simulink library "elementsLibrary"  (R2018a)
settings: Solver=VariableStepAuto  StartTime=0.0  StopTime=10.0  RelTol=1e-3
undefined symbols (not defined in the file): aerodynamics, ascent, avionics, environment, payload, propulsion, pvessel, recovery, rocket, sequencer
libraries: snippetLibrary x43, $bdroot x24, sharedutil x8, theirs_elementsLibrary x3, simulink_extras x1, aerolibutil x1
(part 1 of 4)
settings Model: Creator=Manit  LastModifiedBy=rohan

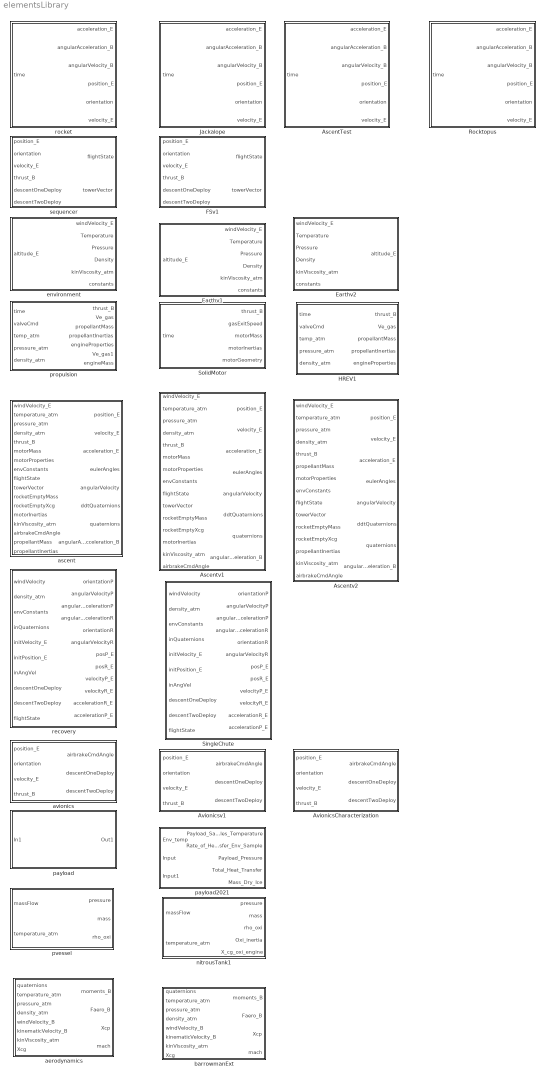
== system elementsLibrary ==
  AscentTest : Subsystem  mask{rocket=rocket}
      settings: MinAlgLoopOccurrences=on
  Ascentv1 : Subsystem  mask{ascent=ascent}
  Ascentv2 : Subsystem  mask{ascent=ascent}
  AvionicsCharacterization : Subsystem  mask{avionics=avionics}
  Avionicsv1 : Subsystem  mask{avionics=avionics}
  Earthv1 : Subsystem  mask{environment=environment}
  Earthv2 : Subsystem  mask{environment=environment}
  FSv1 : Subsystem  mask{sequencer=sequencer}
  HREV1 : Subsystem  mask{propulsion=propulsion}
  Jackalope : Subsystem  mask{rocket=rocket}
      settings: MinAlgLoopOccurrences=on
  Rocktopus : Subsystem  mask{rocket=rocket}
      settings: MinAlgLoopOccurrences=on
  SingleChute : Subsystem  mask{recovery=recovery}
  SolidMotor : Subsystem  mask{propulsion=propulsion}
  aerodynamics : Subsystem  BlockChoice=barrowmanExt
      settings: TemplateBlock=self  MemberBlocks=barrowmanExt
  ascent : Subsystem  BlockChoice=Ascentv1
      settings: TemplateBlock=self  MemberBlocks=Ascentv1,Ascentv2
  avionics : Subsystem  BlockChoice=Avionicsv1
      settings: TemplateBlock=self  MemberBlocks=AvionicsCharacterization,Avionicsv1
  barrowmanExt : Subsystem  mask{aerodynamics=aerodynamics}
  environment : Subsystem  BlockChoice=Earthv1
      settings: TemplateBlock=self  MemberBlocks=Earthv1,Earthv2
  nitrousTank1 : Subsystem  mask{pvessel=pvessel}
  payload : Subsystem  BlockChoice=payload2021
      settings: TemplateBlock=self  MemberBlocks=payload2021
  payload2021 : Subsystem  mask{payload=payload}
  propulsion : Subsystem  BlockChoice=HREV1
      settings: TemplateBlock=self  MemberBlocks=HREV1,SolidMotor
  pvessel : Subsystem  BlockChoice=nitrousTank1
      settings: TemplateBlock=self  MemberBlocks=nitrousTank1
  recovery : Subsystem  BlockChoice=SingleChute
      settings: TemplateBlock=self  MemberBlocks=SingleChute
  rocket : Subsystem  BlockChoice=Jackalope
      settings: TemplateBlock=self  MemberBlocks=Jackalope
  sequencer : Subsystem  BlockChoice=FSv1
      settings: TemplateBlock=self  MemberBlocks=FSv1

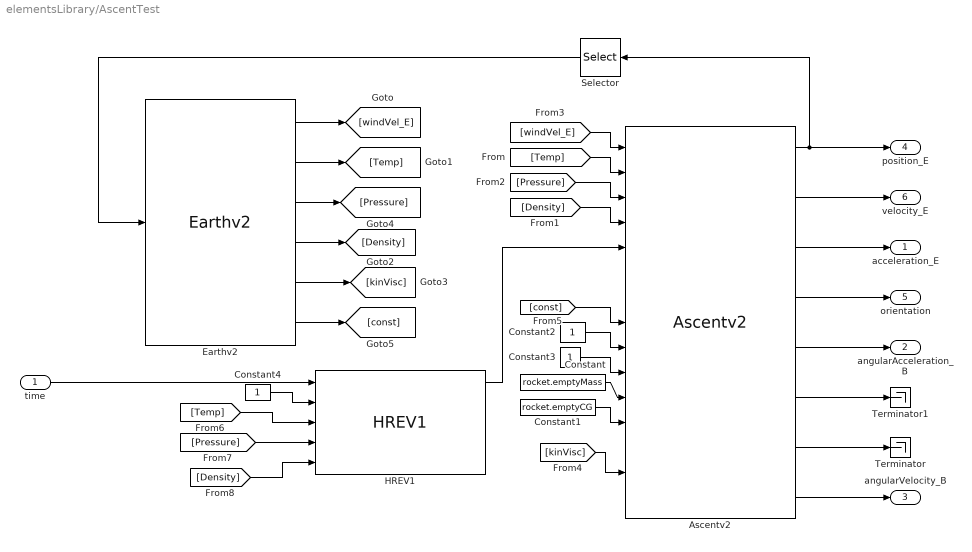
== system elementsLibrary/AscentTest ==
  time : Inport
  Ascentv2 : theirs_elementsLibrary/Ascentv2  ascent=ascent
  Constant : Constant  Value=rocket.emptyMass
  Constant1 : Constant  Value=rocket.emptyCG
  Constant2 : Constant
  Constant3 : Constant
  Constant4 : Constant
  Earthv2 : theirs_elementsLibrary/Earthv2  environment=environment
  HREV1 : theirs_elementsLibrary/HREV1  propulsion=propulsion
  Selector : Selector  InputPortWidth=3  IndexOptions=Index vector (dialog)  Indices=[3]  OutputSizes=1
  Terminator : Terminator
  Terminator1 : Terminator
  acceleration_E : Outport
  angularAcceleration_B : Outport  Port=2
  angularVelocity_B : Outport  Port=3
  position_E : Outport  Port=4
  orientation : Outport  Port=5
  velocity_E : Outport  Port=6
  wires:
  ? -> ?
  time/1 -> HREV1/1
  Ascentv2/1 -> position_E/1, Selector/1
  Selector/1 -> Earthv2/1
  Ascentv2/2 -> velocity_E/1
  Ascentv2/3 -> acceleration_E/1
  Ascentv2/5 -> angularAcceleration_B/1
  Ascentv2/8 -> angularVelocity_B/1
  Ascentv2/4 -> orientation/1
  Ascentv2/7 -> Terminator/1
  Ascentv2/6 -> Terminator1/1
  Earthv2/6 -> [const]
  Earthv2/5 -> [kinVisc]
  Earthv2/4 -> [Density]
  Earthv2/3 -> [Pressure]
  Earthv2/2 -> [Temp]
  Earthv2/1 -> [windVel_E]
  [windVel_E] -> Ascentv2/1
  [Temp] -> Ascentv2/2
  [Pressure] -> Ascentv2/3
  [Density] -> Ascentv2/4
  [const] -> Ascentv2/8
  [kinVisc] -> Ascentv2/14
  HREV1/1 -> Ascentv2/5
  [Temp] -> HREV1/3
  [Pressure] -> HREV1/4
  [Density] -> HREV1/5
  Constant/1 -> Ascentv2/11
  Constant1/1 -> Ascentv2/12
  Constant2/1 -> Ascentv2/9
  Constant3/1 -> Ascentv2/10
  Constant4/1 -> HREV1/2

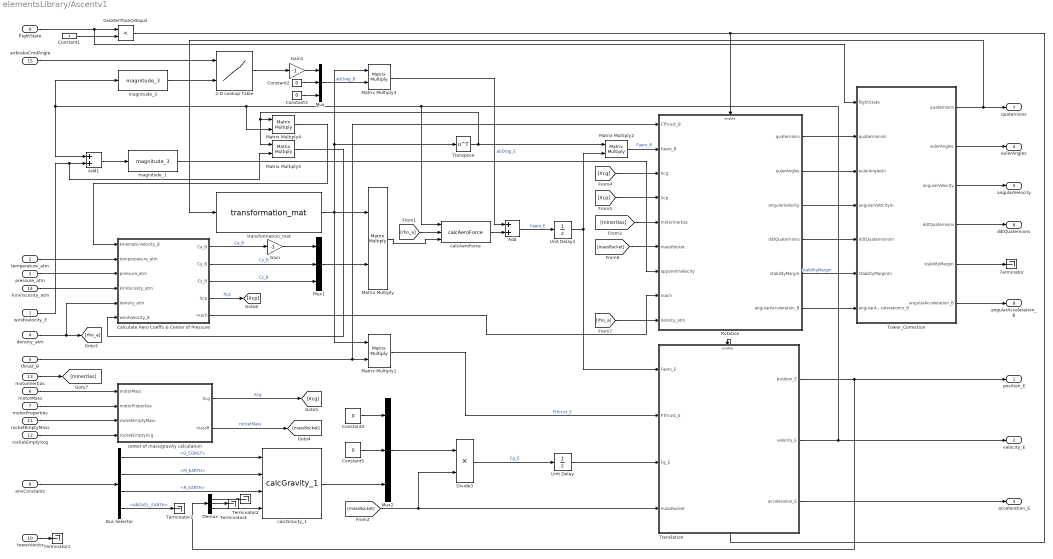
== system elementsLibrary/Ascentv1 ==
  windVelocity_E : Inport
  temperature_atm : Inport  Port=2
  pressure_atm : Inport  Port=3
  density_atm : Inport  Port=4
  thrust_B : Inport  Port=5
  motorMass : Inport  Port=6
  motorProperties : Inport  Port=7
  envConstants : Inport  Port=8
  flightState : Inport  Port=9
  towerVector : Inport  Port=10
  rocketEmptyMass : Inport  Port=11
  rocketEmptyXcg : Inport  Port=12
  motorInertias : Inport  Port=13
  kinViscosity_atm : Inport  Port=14
  airbrakeCmdAngle : Inport  Port=15
  2-D Lookup Table : Lookup_n-D  BreakpointsForDimension1=ascent.aerodynamics.cmdAngleBreakpoints  BreakpointsForDimension2=ascent.aerodynamics.speedBreakpoints  Table=ascent.aerodynamics.increaseInAxialDrag  ExtrapMethod=Clip  UseLastTableValue=on  InternalRulePriority=Speed  RndMeth=Simplest  InputSameDT=on
  Add : Sum
  Add1 : Sum
  Bus Selector : BusSelector  OutputSignals=G_CONST,M_EARTH,R_EARTH,ANGVEL_EARTH
  Calculate Aero Coeffs & Center of Pressure : Subsystem
  Constant1 : Constant  Value=4
  Constant{2..5} (4 alike) : Constant  Value=0
  Demux : Demux  Outputs=3
  Divide3 : Product  Inputs=**
  Gain : Gain  Gain=-1
  Gain1 : Gain  Gain=-1
  GreaterThanOrEqual : RelationalOperator  Operator=<  OutDataTypeStr=boolean  RndMeth=Simplest
  Matrix Multiply{,1..5} (6 alike) : Product  Multiplication=Matrix(*)
  Mux : Mux  Inputs=3
  Mux1 : Mux  Inputs=3
  Mux2 : Mux  Inputs=3
  Rotation : Subsystem
      settings: MinAlgLoopOccurrences=on
  Terminator{,1..4} (5 alike) : Terminator
  Tower_Correction : Subsystem
  Translation : Subsystem
  Transpose : Math  Operator=transpose  SaturateOnIntegerOverflow=on
  Unit Delay : UnitDelay  SampleTime=-1
  Unit Delay1 : UnitDelay  SampleTime=-1
  calcAeroForce : snippetLibrary/aeroSnippets/calcAeroForce  Aref=ascent.aerodynamics.Ar
  calcGravity_1 : snippetLibrary/dynamicsSnippets/calcGravity_1
  center of mass/gravity calculation : Subsystem
  magnitude_1 : snippetLibrary/mathSnippets/magnitude_3
  magnitude_3 : snippetLibrary/mathSnippets/magnitude_3
  transformation_mat : snippetLibrary/mathSnippets/transformation_mat
  position_E : Outport
  velocity_E : Outport  Port=2
  acceleration_E : Outport  Port=3
  eulerAngles : Outport  Port=4
  angularVelocity : Outport  Port=5
  ddtQuaternions : Outport  Port=6
  quaternions : Outport  Port=7
  angularAcceleration_B : Outport  Port=8
  wires:
  pressure_atm/1 -> Calculate Aero Coeffs & Center of Pressure/3(pressure_atm)
  temperature_atm/1 -> Calculate Aero Coeffs & Center of Pressure/2(temperpature_atm)
  density_atm/1 -> Calculate Aero Coeffs & Center of Pressure/5(density_atm), [rho_a]
  windVelocity_E/1 -> Matrix Multiply5/2, Add1/2
  Translation/2(velocity_E) -> velocity_E/1, Matrix Multiply4/2, magnitude_3/1, Add1/1, calcAeroForce/1
  envConstants/1 -> Bus Selector/1
  Bus Selector/4 -> Terminator3/1  "<ANGVEL_EARTH>"
  Bus Selector/1 -> calcGravity_1/1  "<G_CONST>"
  Bus Selector/2 -> calcGravity_1/2  "<M_EARTH>"
  Bus Selector/3 -> calcGravity_1/3  "<R_EARTH>"
  motorMass/1 -> center of mass/gravity calculation/1(motorMass)
  motorProperties/1 -> center of mass/gravity calculation/2(motorProperties)
  rocketEmptyMass/1 -> center of mass/gravity calculation/3(rocketEmptyMass)
  rocketEmptyXcg/1 -> center of mass/gravity calculation/4(rocketEmptyXcg)
  calcAeroForce/1 -> Add/2
  [rho_a] -> calcAeroForce/2
  transformation_mat/1 -> Matrix Multiply/1, Matrix Multiply1/1, Transpose/1, Matrix Multiply3/1
  Mux1/1 -> Matrix Multiply/2
  Matrix Multiply/1 -> calcAeroForce/3
  Calculate Aero Coeffs & Center of Pressure/1(Ca_B) -> Gain/1  "Ca_B"
  Gain/1 -> Mux1/1
  Calculate Aero Coeffs & Center of Pressure/2(Cy_B) -> Mux1/2  "Cy_B"
  Calculate Aero Coeffs & Center of Pressure/3(Cz_B) -> Mux1/3  "Cz_B"
  thrust_B/1 -> Rotation/1(FThrust_B), Matrix Multiply1/2
  Matrix Multiply1/1 -> Translation/2(FThrust_E)  "Fthrust_E"
  Divide3/1 -> Unit Delay/1  "Fg_E"
  Constant5/1 -> Mux2/2
  Mux2/1 -> Divide3/1
  calcGravity_1/1 -> Mux2/3
  Constant4/1 -> Mux2/1
  [massRocket] -> Divide3/2, Translation/4(massRocket)
  center of mass/gravity calculation/2(massR) -> [massRocket]  "rocketMass"
  center of mass/gravity calculation/1(Xcg) -> [Xcg]  "Xcg"
  Calculate Aero Coeffs & Center of Pressure/4(Xcp) -> [Xcp]  "Xcp"
  towerVector/1 -> Terminator1/1
  motorInertias/1 -> [mInertias]
  [mInertias] -> Rotation/5(motorInertias)
  [Xcg] -> Rotation/3(Xcg)
  [Xcp] -> Rotation/4(Xcp)
  Demux/3 -> calcGravity_1/4
  Demux/1 -> Terminator2/1
  Demux/2 -> Terminator4/1
  Matrix Multiply2/1 -> Rotation/2(Faero_B)  "Faero_B"
  Transpose/1 -> Matrix Multiply5/1, Matrix Multiply4/1, Matrix Multiply2/1
  [massRocket] -> Rotation/6(massRocket)
  Rotation/1(quaternions) -> Tower_Correction/2(quaternionsIn)
  airbrakeCmdAngle/1 -> 2-D Lookup Table/1
  flightState/1 -> Tower_Correction/1(flightState), GreaterThanOrEqual/1
  Constant1/1 -> GreaterThanOrEqual/2
  GreaterThanOrEqual/1 -> Rotation/Enable, Translation/Enable
  Mux/1 -> Matrix Multiply3/2  "abDrag_B"
  Constant2/1 -> Mux/2
  Constant3/1 -> Mux/3
  2-D Lookup Table/1 -> Gain1/1
  Gain1/1 -> Mux/1
  magnitude_3/1 -> 2-D Lookup Table/2
  Matrix Multiply3/1 -> Add/1  "abDrag_E"
  Add/1 -> Unit Delay1/1  "Faero_E"
  kinViscosity_atm/1 -> Calculate Aero Coeffs & Center of Pressure/4(kinViscosity_atm)
  Rotation/2(eulerAngles) -> Tower_Correction/3(eulerAnglesIn)
  Rotation/3(angularVelocity) -> Tower_Correction/4(angularVelocityIn)
  Rotation/4(ddtQuaternions) -> Tower_Correction/5(ddtQuaternionsIn)
  Rotation/5(stabilityMargin) -> Tower_Correction/6(stabilityMarginIn)  "stabilityMargin"
  Rotation/6(angularAcceleration_B) -> Tower_Correction/7(angularAccelerationIn_B)
  Translation/1(position_E) -> position_E/1, Demux/1
  Translation/3(acceleration_E) -> acceleration_E/1
  Tower_Correction/1(quaternions) -> quaternions/1, transformation_mat/1
  Tower_Correction/2(eulerAngles) -> eulerAngles/1
  Tower_Correction/3(angularVelocity) -> angularVelocity/1
  Tower_Correction/4(ddtQuaternions) -> ddtQuaternions/1
  Tower_Correction/5(stabilityMargin) -> Terminator/1
  Tower_Correction/6(angularAcceleration_B) -> angularAcceleration_B/1
  Unit Delay/1 -> Translation/3(Fg_E)
  Unit Delay1/1 -> Translation/1(Faero_E), Matrix Multiply2/2
  magnitude_1/1 -> Rotation/7(apparentVelocity)
  Calculate Aero Coeffs & Center of Pressure/5(mach) -> Rotation/8(mach)
  Add1/1 -> magnitude_1/1
  [rho_a] -> Rotation/9(density_atm)
  Matrix Multiply4/1 -> Calculate Aero Coeffs & Center of Pressure/1(kinematicVelocity_B)
  Matrix Multiply5/1 -> Calculate Aero Coeffs & Center of Pressure/6(windVelocity_B)

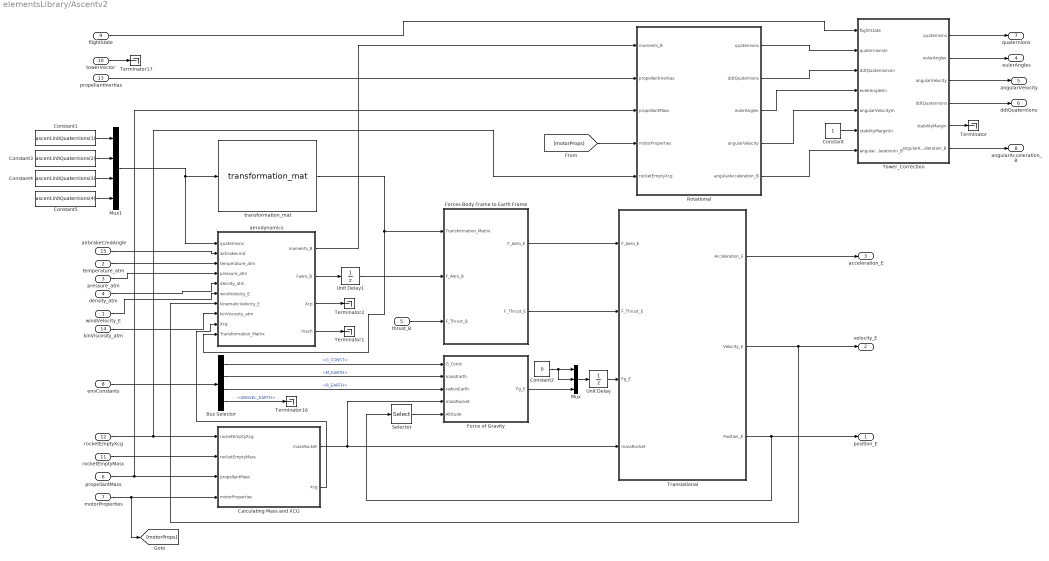
== system elementsLibrary/Ascentv2 ==
  windVelocity_E : Inport
  temperature_atm : Inport  Port=2
  pressure_atm : Inport  Port=3
  density_atm : Inport  Port=4
  thrust_B : Inport  Port=5
  propellantMass : Inport  Port=6
  motorProperties : Inport  Port=7
  envConstants : Inport  Port=8
  flightState : Inport  Port=9
  towerVector : Inport  Port=10
  rocketEmptyMass : Inport  Port=11
  rocketEmptyXcg : Inport  Port=12
  propellantInertias : Inport  Port=13
  kinViscosity_atm : Inport  Port=14
  airbrakeCmdAngle : Inport  Port=15
  Bus Selector : BusSelector  OutputSignals=G_CONST,M_EARTH,R_EARTH,ANGVEL_EARTH
  Calculating Mass and XCG : Subsystem
  Constant : Constant
  Constant1 : Constant  Value=ascent.initQuaternions(1)
  Constant2 : Constant  Value=0
  Constant3 : Constant  Value=ascent.initQuaternions(2)
  Constant4 : Constant  Value=ascent.initQuaternions(3)
  Constant5 : Constant  Value=ascent.initQuaternions(4)
  Force of Gravity : Subsystem
  Forces Body Frame to Earth Frame : Subsystem
  Mux : Mux  Inputs=3
  Mux1 : Mux
  Rotational : Subsystem
  Selector : Selector  InputPortWidth=3  IndexOptions=Index vector (dialog)  Indices=[3]  OutputSizes=1
  Terminator{,1..2,16..17} (5 alike) : Terminator
  Tower_Correction : Subsystem
  "Translational " : Subsystem
  Unit Delay : UnitDelay  SampleTime=-1
  Unit Delay1 : UnitDelay  SampleTime=-1
  aerodynamics : Subsystem
  transformation_mat : snippetLibrary/mathSnippets/transformation_mat
  position_E : Outport
  velocity_E : Outport  Port=2
  acceleration_E : Outport  Port=3
  eulerAngles : Outport  Port=4
  angularVelocity : Outport  Port=5
  ddtQuaternions : Outport  Port=6
  quaternions : Outport  Port=7
  angularAcceleration_B : Outport  Port=8
  wires:
  Force of Gravity/1(Fg_E) -> Mux/3
  thrust_B/1 -> Forces Body Frame to Earth Frame/3(F_Thrust_B)
  Bus Selector/3 -> Force of Gravity/3(radiusEarth)  "<R_EARTH>"
  propellantMass/1 -> Calculating Mass and XCG/3(propellantMass), Rotational/3(propellantMass)
  Constant2/1 -> Mux/1, Mux/2
  rocketEmptyXcg/1 -> Calculating Mass and XCG/1(rocketEmptyXcg), Rotational/5(rocketEmptyXcg)
  Calculating Mass and XCG/1(massRocket) -> Force of Gravity/4(massRocket), "Translational "/4(massRocket)
  Forces Body Frame to Earth Frame/2(F_Thrust_E) -> "Translational "/2(F_Thrust_E)
  towerVector/1 -> Terminator17/1
  Bus Selector/4 -> Terminator16/1  "<ANGVEL_EARTH>"
  flightState/1 -> Tower_Correction/1(flightState)
  Bus Selector/2 -> Force of Gravity/2(massEarth)  "<M_EARTH>"
  rocketEmptyMass/1 -> Calculating Mass and XCG/2(rocketEmptyMass)
  pressure_atm/1 -> aerodynamics/4(pressure_atm)
  Selector/1 -> Force of Gravity/5(Altitude)
  Forces Body Frame to Earth Frame/1(F_Aero_E) -> "Translational "/1(F_Aero_E)
  motorProperties/1 -> [motorProps], Calculating Mass and XCG/4(motorProperties)
  airbrakeCmdAngle/1 -> aerodynamics/2(airbrakecmd)
  Bus Selector/1 -> Force of Gravity/1(G_Const)  "<G_CONST>"
  "Translational "/1(Acceleration_E) -> acceleration_E/1
  envConstants/1 -> Bus Selector/1
  propellantInertias/1 -> Rotational/2(propellentInertias)
  "Translational "/3(Position_E) -> position_E/1, Selector/1
  Calculating Mass and XCG/2(Xcg) -> aerodynamics/9(Xcg)
  "Translational "/2(Velocity_E) -> velocity_E/1, aerodynamics/7(kinematicVelocity_E)
  transformation_mat/1 -> Forces Body Frame to Earth Frame/1(Transformation_Matrix), aerodynamics/10(Transformation_Matrix)
  kinViscosity_atm/1 -> aerodynamics/8(kinViscosity_atm)
  windVelocity_E/1 -> aerodynamics/6(windVelocity_E)
  density_atm/1 -> aerodynamics/5(density_atm)
  temperature_atm/1 -> aerodynamics/3(temperature_atm)
  aerodynamics/1(moments_B) -> Rotational/1(moments_B)
  aerodynamics/3(Xcp) -> Terminator2/1
  aerodynamics/4(mach) -> Terminator1/1
  [motorProps] -> Rotational/4(motorProperties)
  Mux/1 -> Unit Delay/1
  Unit Delay/1 -> "Translational "/3(Fg_E)
  aerodynamics/2(Faero_B) -> Unit Delay1/1
  Unit Delay1/1 -> Forces Body Frame to Earth Frame/2(F_Aero_B)
  Constant/1 -> Tower_Correction/6(stabilityMarginIn)
  Rotational/5(angularAcceleration_B) -> Tower_Correction/7(angularAccelerationIn_B)
  Rotational/4(angularVelocity) -> Tower_Correction/5(angularVelocityIn)
  Rotational/3(eulerAngles) -> Tower_Correction/4(eulerAnglesIn)
  Rotational/2(ddtQuaternions) -> Tower_Correction/3(ddtQuaternionsIn)
  Tower_Correction/6(angularAcceleration_B) -> angularAcceleration_B/1
  Tower_Correction/3(angularVelocity) -> angularVelocity/1
  Tower_Correction/4(ddtQuaternions) -> ddtQuaternions/1
  Tower_Correction/2(eulerAngles) -> eulerAngles/1
  Tower_Correction/1(quaternions) -> quaternions/1
  Tower_Correction/5(stabilityMargin) -> Terminator/1
  Rotational/1(quaternions) -> Tower_Correction/2(quaternionsIn)
  Constant5/1 -> Mux1/4
  Constant3/1 -> Mux1/2
  Constant1/1 -> Mux1/1
  Constant4/1 -> Mux1/3
  Mux1/1 -> transformation_mat/1, aerodynamics/1(quaternions)

== system elementsLibrary/AvionicsCharacterization ==
  position_E : Inport
  orientation : Inport  Port=2
  velocity_E : Inport  Port=3
  thrust_B : Inport  Port=4
  Constant : Constant  Value=avionics.airbrakeDeploySpeed
  Constant1 : Constant  Value=avionics.airbrakeDeployCmd
  Constant2 : Constant  Value=avionics.descentTwoDeployAltitude
  Demux1 : Demux  Outputs=3
  Demux2 : Demux  Outputs=3
  MATLAB Function : MATLAB Function  TreatAsAtomicUnit=on
  Terminator{1..5} (5 alike) : Terminator
  Unit Delay : UnitDelay  InitialCondition=false  SampleTime=-1
  Unit Delay1 : UnitDelay  InitialCondition=false  SampleTime=-1
  Unit Delay2 : UnitDelay  InitialCondition=false  SampleTime=-1
  magnitude_1 : snippetLibrary/mathSnippets/magnitude_3
  magnitude_3 : snippetLibrary/mathSnippets/magnitude_3
  airbrakeCmdAngle : Outport
  descentOneDeploy : Outport  Port=2
  descentTwoDeploy : Outport  Port=3
  wires:
  thrust_B/1 -> magnitude_3/1
  velocity_E/1 -> Demux2/1, magnitude_1/1
  orientation/1 -> Terminator1/1
  position_E/1 -> Demux1/1
  MATLAB Function/1(airbrakeCmdAngle) -> Unit Delay2/1  "airbrakeCmdAngle"
  MATLAB Function/2(deploy1) -> Unit Delay1/1  "descentOneDeploy"
  MATLAB Function/3(deploy2) -> Unit Delay/1  "descentTwoDeploy"
  magnitude_1/1 -> MATLAB Function/2(velMag)
  Demux1/3 -> MATLAB Function/1(posZ_E)
  Demux1/1 -> Terminator2/1
  Demux1/2 -> Terminator3/1
  Constant/1 -> MATLAB Function/5(airbrakeDeploySpeed)
  Constant1/1 -> MATLAB Function/6(airbrakeDeployCmd)
  Constant2/1 -> MATLAB Function/7(descentTwoDeployAltitude)
  Demux2/3 -> MATLAB Function/3(velZ_E)
  Demux2/1 -> Terminator4/1
  Demux2/2 -> Terminator5/1
  Unit Delay/1 -> MATLAB Function/9(prevDeploy2), descentTwoDeploy/1
  magnitude_3/1 -> MATLAB Function/4(thurstMag_B)
  Unit Delay1/1 -> MATLAB Function/8(prevDeploy1), descentOneDeploy/1
  Unit Delay2/1 -> airbrakeCmdAngle/1

== system elementsLibrary/Avionicsv1 ==
  position_E : Inport
  orientation : Inport  Port=2
  velocity_E : Inport  Port=3
  thrust_B : Inport  Port=4
  airbrakeCmdAngle : Outport
  descentOneDeploy : Outport  Port=2
  descentTwoDeploy : Outport  Port=3

== system elementsLibrary/Earthv1 ==
  altitude_E : Inport
  1-D Lookup Table : Lookup_n-D  NumberOfTableDimensions=1  BreakpointsForDimension1=environment.altiBreakpoints  Table=environment.dynamicViscosityAir  ExtrapMethod=Clip  UseLastTableValue=on  InternalRulePriority=Speed  RndMeth=Simplest  InputSameDT=on
  Abs : Abs
  Bus Creator : BusCreator  Inputs=4
  Constant : Constant  Value=environment.RADIUS_EARTH
  Constant1 : Constant  Value=environment.MASS_EARTH
  Constant2 : Constant  Value=environment.ANGULARVELOCITY_EARTH
  Constant3 : Constant  Value=environment.GRAVITATION_CONST
  Constant4 : Constant  Value=0
  Cos : Trigonometry  Operator=cos
  Divide : Product  Inputs=/*
  MATLAB Function : MATLAB Function  TreatAsAtomicUnit=on
  Multiply : Product
  Multiply1 : Product
  Mux : Mux  Inputs=3
  Sin : Trigonometry
  Terminator : Terminator
  Wind Velocity Calculation : Subsystem
  encoded wind direction : Constant  Value=environment.referenceWindAngle
  windVelocity_E : Outport
  Temperature : Outport  Port=2
  Pressure : Outport  Port=3
  Density : Outport  Port=4
  kinViscosity_atm : Outport  Port=5
  constants : Outport  Port=6
  wires:
  MATLAB Function/3(density) -> Divide/1, Density/1  "atmos_density"
  MATLAB Function/2(pressure) -> Pressure/1  "atmos_pressure"
  Wind Velocity Calculation/1(Out1) -> Multiply1/1, Multiply/1  "windspeed"
  altitude_E/1 -> Wind Velocity Calculation/1(In1), Wind Velocity Calculation/2(Altitude), 1-D Lookup Table/1, MATLAB Function/1(altitude)
  MATLAB Function/1(temperature) -> Temperature/1  "atmos_temperature"
  Constant/1 -> Bus Creator/1  "R_EARTH"
  Constant1/1 -> Bus Creator/2  "M_EARTH"
  Constant2/1 -> Bus Creator/3  "ANGVEL_EARTH"
  Constant3/1 -> Bus Creator/4  "G_CONST"
  encoded wind direction/1 -> [windAngle]
  Multiply1/1 -> Mux/2
  Multiply/1 -> Mux/1
  Constant4/1 -> Mux/3
  Mux/1 -> Abs/1  "windvelocity_E"
  [windAngle] -> Sin/1, Cos/1
  Cos/1 -> Multiply/2
  Sin/1 -> Multiply1/2
  Bus Creator/1 -> constants/1
  1-D Lookup Table/1 -> Terminator/1, Divide/2  "dynamicViscosity"
  Divide/1 -> kinViscosity_atm/1  "kinViscosity"
  Abs/1 -> windVelocity_E/1

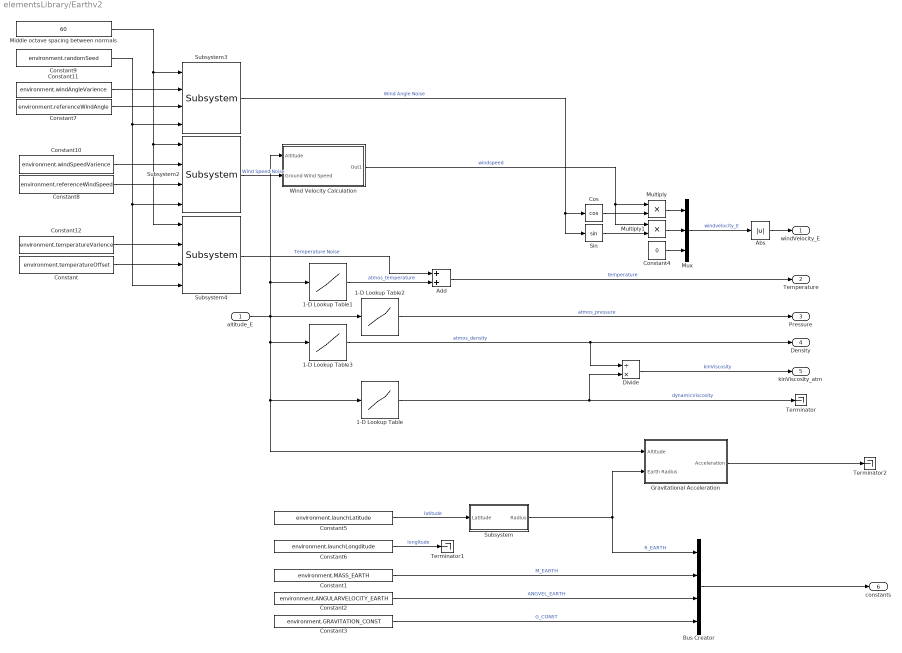
== system elementsLibrary/Earthv2 ==
  altitude_E : Inport
  1-D Lookup Table : Lookup_n-D  NumberOfTableDimensions=1  BreakpointsForDimension1=environment.altiBreakpoints  Table=environment.dynamicViscosityAir  ExtrapMethod=Clip  UseLastTableValue=on  InternalRulePriority=Speed  RndMeth=Simplest  InputSameDT=on
  1-D Lookup Table1 : Lookup_n-D  NumberOfTableDimensions=1  BreakpointsForDimension1=environment.altiBreakpoints  Table=environment.temperatureAir  ExtrapMethod=Clip  UseLastTableValue=on  InternalRulePriority=Speed  RndMeth=Simplest  InputSameDT=on
  1-D Lookup Table2 : Lookup_n-D  NumberOfTableDimensions=1  BreakpointsForDimension1=environment.altiBreakpoints  Table=environment.pressureAir  ExtrapMethod=Clip  UseLastTableValue=on  InternalRulePriority=Speed  RndMeth=Simplest  InputSameDT=on
  1-D Lookup Table3 : Lookup_n-D  NumberOfTableDimensions=1  BreakpointsForDimension1=environment.altiBreakpoints  Table=environment.densityAir  ExtrapMethod=Clip  UseLastTableValue=on  InternalRulePriority=Speed  RndMeth=Simplest  InputSameDT=on
  Abs : Abs
  Add : Sum
  Bus Creator : BusCreator  Inputs=4
  Constant : Constant  Value=environment.temperatureOffset
  Constant1 : Constant  Value=environment.MASS_EARTH
  Constant10 : Constant  Value=environment.windSpeedVarience
  Constant11 : Constant  Value=environment.windAngleVarience
  Constant12 : Constant  Value=environment.temperatureVarience
  Constant2 : Constant  Value=environment.ANGULARVELOCITY_EARTH
  Constant3 : Constant  Value=environment.GRAVITATION_CONST
  Constant4 : Constant  Value=0
  Constant5 : Constant  Value=environment.launchLatitude
  Constant6 : Constant  Value=environment.launchLongditude
  Constant7 : Constant  Value=environment.referenceWindAngle
  Constant8 : Constant  Value=environment.referenceWindSpeed
  Constant9 : Constant  Value=environment.randomSeed
  Cos : Trigonometry  Operator=cos
  Divide : Product  Inputs=/*
  Gravitational Acceleration : Subsystem
  Middle octave spacing between normals : Constant  Value=60
  Multiply : Product
  Multiply1 : Product
  Mux : Mux  Inputs=3
  Sin : Trigonometry
  Subsystem : Subsystem
  Subsystem2 : snippetLibrary/environmentSnippets/Subsystem
  Subsystem3 : snippetLibrary/environmentSnippets/Subsystem
  Subsystem4 : snippetLibrary/environmentSnippets/Subsystem
  Terminator : Terminator
  Terminator1 : Terminator
  Terminator2 : Terminator
  Wind Velocity Calculation : Subsystem
  windVelocity_E : Outport
  Temperature : Outport  Port=2
  Pressure : Outport  Port=3
  Density : Outport  Port=4
  kinViscosity_atm : Outport  Port=5
  constants : Outport  Port=6
  wires:
  Constant9/1 -> Subsystem4/4, Subsystem2/4, Subsystem3/4
  Constant12/1 -> Subsystem4/2
  Constant11/1 -> Subsystem3/2
  Constant10/1 -> Subsystem2/2
  Middle octave spacing between normals/1 -> Subsystem3/1, Subsystem2/1, Subsystem4/1
  Constant8/1 -> Subsystem2/3
  Constant7/1 -> Subsystem3/3
  Constant/1 -> Subsystem4/3
  Subsystem4/1 -> Add/1  "Temperature Noise"
  Subsystem3/1 -> Cos/1, Sin/1  "Wind Angle Noise"
  Subsystem2/1 -> Wind Velocity Calculation/2(Ground Wind Speed)  "Wind Speed Noise"
  Add/1 -> Temperature/1  "temperature"
  Subsystem/1(Radius) -> Gravitational Acceleration/2(Earth Radius), Bus Creator/1  "R_EARTH"
  Gravitational Acceleration/1(Acceleration) -> Terminator2/1
  Constant5/1 -> Subsystem/1(Latitude)  "latitude"
  Constant6/1 -> Terminator1/1  "longitude"
  altitude_E/1 -> 1-D Lookup Table3/1, 1-D Lookup Table/1, Gravitational Acceleration/1(Altitude), 1-D Lookup Table1/1, Wind Velocity Calculation/1(Altitude), 1-D Lookup Table2/1
  Abs/1 -> windVelocity_E/1
  Divide/1 -> kinViscosity_atm/1  "kinViscosity"
  1-D Lookup Table/1 -> Divide/2, Terminator/1  "dynamicViscosity"
  Bus Creator/1 -> constants/1
  Sin/1 -> Multiply1/2
  Cos/1 -> Multiply/2
  Mux/1 -> Abs/1  "windvelocity_E"
  Constant4/1 -> Mux/3
  Multiply/1 -> Mux/1
  Multiply1/1 -> Mux/2
  Constant3/1 -> Bus Creator/4  "G_CONST"
  Constant2/1 -> Bus Creator/3  "ANGVEL_EARTH"
  Constant1/1 -> Bus Creator/2  "M_EARTH"
  1-D Lookup Table1/1 -> Add/2  "atmos_temperature"
  Wind Velocity Calculation/1(Out1) -> Multiply/1, Multiply1/1  "windspeed"
  1-D Lookup Table2/1 -> Pressure/1  "atmos_pressure"
  1-D Lookup Table3/1 -> Density/1, Divide/1  "atmos_density"

== system elementsLibrary/FSv1 ==
  position_E : Inport
  orientation : Inport  Port=2
  velocity_E : Inport  Port=3
  thrust_B : Inport  Port=4
  descentOneDeploy : Inport  Port=5
  descentTwoDeploy : Inport  Port=6
  Demux1 : Demux  Outputs=3
  Demux2 : Demux  Outputs=3
  Demux4 : Demux  Outputs=3
  Length of Launch Tower1 : Constant  Value=sequencer.launchTower(1)
  Length of Launch Tower2 : Constant  Value=sequencer.launchTower(2)
  Length of Launch Tower3 : Constant  Value=sequencer.launchTower(3)
  MATLAB Function : MATLAB Function  TreatAsAtomicUnit=on
  Mux : Mux  Inputs=3
  Stop Simulation : Stop
  Unit Delay : UnitDelay  InitialCondition=sequencer.initialFlightState  SampleTime=-1
  magnitude3_1 : snippetLibrary/mathSnippets/magnitude_3
  magnitude3_3 : snippetLibrary/mathSnippets/magnitude_3
  magnitude_3 : snippetLibrary/mathSnippets/magnitude_3
  flightState : Outport
  towerVector : Outport  Port=2
  wires:
  position_E/1 -> magnitude3_1/1, Demux1/1
  MATLAB Function/1(flightState) -> Unit Delay/1  "flightState"
  thrust_B/1 -> magnitude_3/1
  Demux1/1 -> MATLAB Function/3(posX_E)
  Demux1/2 -> MATLAB Function/4(posY_E)
  Demux1/3 -> MATLAB Function/5(posZ_E)
  orientation/1 -> Demux2/1
  Length of Launch Tower1/1 -> Mux/1
  Length of Launch Tower2/1 -> Mux/2
  Length of Launch Tower3/1 -> Mux/3
  Mux/1 -> magnitude3_3/1, towerVector/1
  Demux2/2 -> MATLAB Function/7(pitch)
  Demux2/3 -> MATLAB Function/8(yaw)
  Demux2/1 -> MATLAB Function/6(roll)
  Unit Delay/1 -> MATLAB Function/15(prevFlightState), flightState/1
  magnitude3_1/1 -> MATLAB Function/2(posMag)
  Demux4/2 -> MATLAB Function/10(velY_E)
  Demux4/1 -> MATLAB Function/9(velX_E)
  Demux4/3 -> MATLAB Function/11(velZ_E)
  velocity_E/1 -> Demux4/1
  [towerLen] -> MATLAB Function/1(towerLen)
  magnitude_3/1 -> MATLAB Function/14(thurstMag_B)
  magnitude3_3/1 -> [towerLen]
  descentOneDeploy/1 -> MATLAB Function/12(descentOneDeploy)
  descentTwoDeploy/1 -> MATLAB Function/13(descentTwoDeploy)
  MATLAB Function/2(stop) -> Stop Simulation/1

== system elementsLibrary/HREV1 ==
  time : Inport
  valveCmd : Inport  Port=2
  temp_atm : Inport  Port=3
  pressure_atm : Inport  Port=4
  "density_atm " : Inport  Port=5
  Add1 : Sum
  Bus Creator : BusCreator  Inputs=2
  Chamber_Ballistics : Subsystem
  Injecter : Subsystem
  Nozzle : Subsystem
  Propellant_Mass : Subsystem
  Terminator{,1..8} (9 alike) : Terminator
  Unit Delay : UnitDelay  SampleTime=-1
  Unit Delay1 : UnitDelay  InitialCondition=101.325  SampleTime=-1
  X_grain_to_engine : Constant  Value=propulsion.X_TanktoGrain
  X_nose_to_engine : Constant  Value=propulsion.X_GM
  cg_propellent_engine : Subsystem
  nitrousTank1 : $bdroot/nitrousTank1  pvessel=propulsion.pvessel
  parallel_axis_propellent : Subsystem
  thrust_B : Outport
  Ve_gas : Outport  Port=2
  propellantMass : Outport  Port=3
  propellantInertias : Outport  Port=4
  engineProperties : Outport  Port=5
  wires:
  time/1 -> Terminator/1
  valveCmd/1 -> Terminator1/1
  pressure_atm/1 -> Nozzle/4(P_atm)
  Chamber_Ballistics/2(mdot_total) -> Nozzle/1(mdot)  "mdot_total"
  Chamber_Ballistics/3(Pc) -> Unit Delay1/1  "Pchamber"
  Chamber_Ballistics/4(Tc) -> Nozzle/3(Tc)  "Tchamber"
  Chamber_Ballistics/1(mdot_fuel) -> Terminator5/1  "mdot_fuel"
  Chamber_Ballistics/5(rdot_fuel) -> Terminator6/1  "rdot_fuel"
  nitrousTank1/2 -> Injecter/4(mass_oxi), cg_propellent_engine/4(mass_oxi), parallel_axis_propellent/1(mass_oxi), Propellant_Mass/1(mass_oxi)
  Chamber_Ballistics/6(massFlux_oxi) -> Terminator7/1  "Gox"
  Chamber_Ballistics/7(OF_ratio) -> Terminator8/1  "OF_ratio"
  Nozzle/4(charV) -> Unit Delay/1  "cStar"
  Unit Delay/1 -> Chamber_Ballistics/2(cStar)
  "density_atm "/1 -> Terminator3/1
  Nozzle/2(V_exit) -> Ve_gas/1  "Ve_gas"
  Nozzle/1(thrust_B) -> thrust_B/1  "thrust_B"
  Nozzle/3(mach_exit) -> Terminator4/1  "mach_exit"
  Propellant_Mass/1(massProp) -> propellantMass/1  "propellant_mass"
  Unit Delay1/1 -> Injecter/2(Chamber_pressure), Nozzle/2(Pc)
  Chamber_Ballistics/8(mass_fuel) -> cg_propellent_engine/2(mass_fuel), parallel_axis_propellent/6(mass_fuel), Propellant_Mass/2(mass_fuel)  "mass_fuel"
  X_grain_to_engine/1 -> Add1/2
  Chamber_Ballistics/10(X_cg_fuel) -> Add1/1
  Add1/1 -> cg_propellent_engine/1(X_cg_fuel_engine), parallel_axis_propellent/5(X_cg_fuel_engine)  "X_cg_fuel_engine"
  nitrousTank1/5 -> cg_propellent_engine/3(X_cg_oxi_engine), parallel_axis_propellent/3(X_cg_oxi_engine)
  cg_propellent_engine/1(cg_prop_engine) -> parallel_axis_propellent/8(X_cg_prop_engine), Bus Creator/2  "x_cg_B"
  parallel_axis_propellent/1(Propellent_inertia) -> propellantInertias/1
  nitrousTank1/4 -> parallel_axis_propellent/2(Oxi_inertia)
  Chamber_Ballistics/9(Fuel_inertia) -> parallel_axis_propellent/4(Fuel_inertia)
  X_nose_to_engine/1 -> Bus Creator/1, parallel_axis_propellent/7(X_nose_to_engine)  "x_gm_B"
  Bus Creator/1 -> engineProperties/1
  Injecter/1(mdot_oxi) -> nitrousTank1/1, Chamber_Ballistics/1(mdot_oxi)  "mdot_oxi"
  nitrousTank1/1 -> Injecter/1("Tank_pressure ")
  nitrousTank1/3 -> Injecter/3(density_oxi)
  temp_atm/1 -> nitrousTank1/2

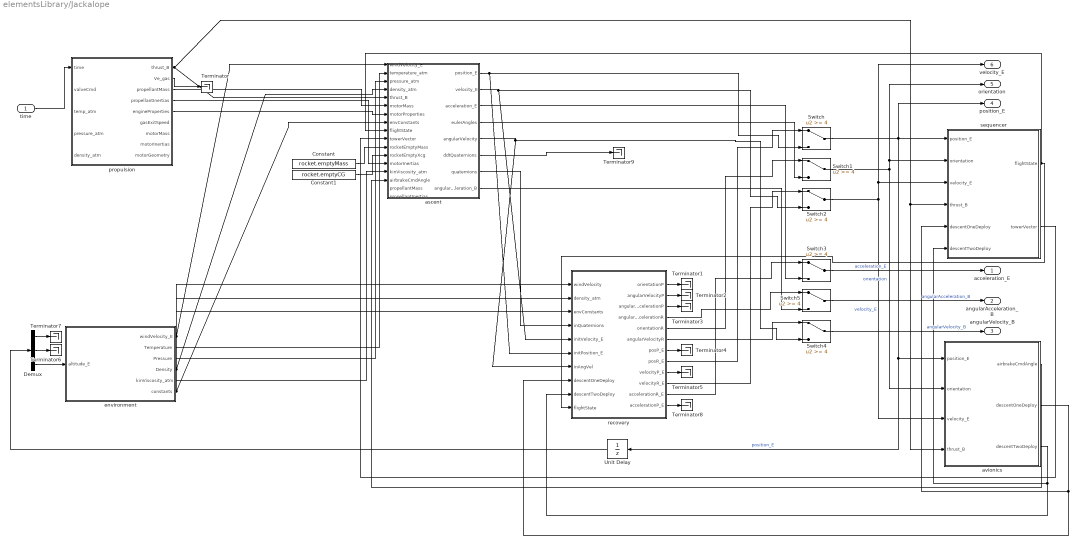
== system elementsLibrary/Jackalope ==
  time : Inport
  Constant : Constant  Value=rocket.emptyMass
  Constant1 : Constant  Value=rocket.emptyCG
  Demux : Demux  Outputs=3
  Switch{,1..5} (6 alike) : Switch  Threshold=4
  Terminator{,1..9} (10 alike) : Terminator
  Unit Delay : UnitDelay  SampleTime=-1
  ascent : Subsystem  BlockChoice=Ascentv1
      settings: AttributesFormatString=%<BlockChoice>  TemplateBlock=elementsLibrary/ascent  MemberBlocks=Ascentv1,Ascentv2
  avionics : Subsystem  BlockChoice=AvionicsCharacterization
      link override AvionicsCharacterization: avionics=rocket.avionics
      link override Avionicsv1: avionics=rocket.avionics
      settings: AttributesFormatString=%<BlockChoice>  TemplateBlock=elementsLibrary/avionics  MemberBlocks=AvionicsCharacterization,Avionicsv1
  environment : Subsystem  BlockChoice=Earthv1
      link override Earthv1: environment=rocket.environment
      settings: AttributesFormatString=%<BlockChoice>  TemplateBlock=elementsLibrary/environment  MemberBlocks=Earthv1,Earthv2
  propulsion : Subsystem  BlockChoice=SolidMotor
      link override SolidMotor: propulsion=rocket.propulsion
      settings: AttributesFormatString=%<BlockChoice>  TemplateBlock=elementsLibrary/propulsion  MemberBlocks=HREV1,SolidMotor
  recovery : Subsystem  BlockChoice=SingleChute
      link override SingleChute: recovery=rocket.recovery
      settings: AttributesFormatString=%<BlockChoice>  TemplateBlock=elementsLibrary/recovery  MemberBlocks=SingleChute
  sequencer : Subsystem  BlockChoice=FSv1
      link override FSv1: sequencer=rocket.sequencer
      settings: AttributesFormatString=%<BlockChoice>  TemplateBlock=elementsLibrary/sequencer  MemberBlocks=FSv1
  acceleration_E : Outport
  angularAcceleration_B : Outport  Port=2
  angularVelocity_B : Outport  Port=3
  position_E : Outport  Port=4
  orientation : Outport  Port=5
  velocity_E : Outport  Port=6
  wires:
  time/1 -> propulsion/1(time)
  Switch/1 -> sequencer/1(position_E), avionics/1(position_E), Unit Delay/1, position_E/1  "position_E"
  Switch1/1 -> avionics/2(orientation), sequencer/2(orientation), orientation/1  "orientation"
  Switch2/1 -> avionics/3(velocity_E), sequencer/3(velocity_E), velocity_E/1  "velocity_E"
  recovery/8(posR_E) -> Switch/1
  recovery/10(velocityR_E) -> Switch2/1
  ascent/4(eulerAngles) -> Switch1/3
  recovery/5(orientationR) -> Switch1/1
  environment/4(Density) -> ascent/4(density_atm), recovery/2(density_atm)
  environment/6(constants) -> ascent/8(envConstants), recovery/3(envConstants)
  environment/3(Pressure) -> ascent/3(pressure_atm)
  environment/2(Temperature) -> ascent/2(temperature_atm)
  environment/1(windVelocity_E) -> ascent/1(windVelocity_E), recovery/1(windVelocity)
  propulsion/3(propellantMass) -> ascent/6(motorMass)
  propulsion/4(propellantInertias) -> ascent/13(motorInertias)
  propulsion/1(thrust_B) -> ascent/5(thrust_B), sequencer/4(thrust_B), avionics/4(thrust_B)
  propulsion/5(engineProperties) -> ascent/7(motorProperties)
  propulsion/2(Ve_gas) -> Terminator/1
  sequencer/2(towerVector) -> ascent/10(towerVector)
  ascent/5(angularVelocity) -> recovery/7(inAngVel), Switch4/3
  ascent/1(position_E) -> Switch/3, recovery/6(initPosition_E)
  ascent/2(velocity_E) -> Switch2/3, recovery/5(initVelocity_E)
  recovery/2(angularVelocityP) -> Terminator2/1
  recovery/1(orientationP) -> Terminator1/1
  recovery/3(angularAccelerationP) -> Terminator3/1
  recovery/7(posP_E) -> Terminator4/1
  recovery/9(velocityP_E) -> Terminator5/1
  ascent/3(acceleration_E) -> Switch3/3
  ascent/7(quaternions) -> recovery/4(inQuaternions)
  Demux/3 -> environment/1(altitude_E)
  Demux/2 -> Terminator6/1
  Demux/1 -> Terminator7/1
  recovery/12(accelerationP_E) -> Terminator8/1
  recovery/11(accelerationR_E) -> Switch3/1
  Switch3/1 -> acceleration_E/1  "acceleration_E"
  recovery/4(angularAccelerationR) -> Switch5/1
  recovery/6(angularVelocityR) -> Switch4/1
  ascent/8(angularAcceleration_B) -> Switch5/3
  Switch5/1 -> angularAcceleration_B/1  "angularAcceleration_B"
  Switch4/1 -> angularVelocity_B/1  "angularVelocity_B"
  ascent/6(ddtQuaternions) -> Terminator9/1
  Constant/1 -> ascent/11(rocketEmptyMass)
  Constant1/1 -> ascent/12(rocketEmptyXcg)
  environment/5(kinViscosity_atm) -> ascent/14(kinViscosity_atm)
  avionics/3(descentTwoDeploy) -> recovery/9(descentTwoDeploy), sequencer/6(descentTwoDeploy)
  avionics/2(descentOneDeploy) -> sequencer/5(descentOneDeploy), recovery/8(descentOneDeploy)
  avionics/1(airbrakeCmdAngle) -> ascent/15(airbrakeCmdAngle)
  Unit Delay/1 -> Demux/1
  sequencer/1(flightState) -> ascent/9(flightState), recovery/10(flightState)

== system elementsLibrary/Rocktopus ==
  time : Inport
  Constant : Constant  Value=rocket.emptyMass
  Constant1 : Constant  Value=rocket.emptyCG
  Demux : Demux  Outputs=3
  Switch{,1..5} (6 alike) : Switch  Threshold=4
  Terminator{,1..9} (10 alike) : Terminator
  Unit Delay : UnitDelay  SampleTime=-1
  ascent : Subsystem  BlockChoice=Ascentv2
      link override Ascentv2: ascent=rocket.ascent
      settings: AttributesFormatString=%<BlockChoice>  TemplateBlock=elementsLibrary/ascent  MemberBlocks=Ascentv1,Ascentv2
  avionics : Subsystem  BlockChoice=AvionicsCharacterization
      link override AvionicsCharacterization: avionics=rocket.avionics
      link override Avionicsv1: avionics=rocket.avionics
      settings: AttributesFormatString=%<BlockChoice>  TemplateBlock=elementsLibrary/avionics  MemberBlocks=AvionicsCharacterization,Avionicsv1
  environment : Subsystem  BlockChoice=Earthv1
      link override Earthv1: environment=rocket.environment
      settings: AttributesFormatString=%<BlockChoice>  TemplateBlock=elementsLibrary/environment  MemberBlocks=Earthv1,Earthv2
  propulsion : Subsystem  BlockChoice=HREV1
      link override HREV1: propulsion=rocket.propulsion
      link override SolidMotor: propulsion=rocket.propulsion
      settings: AttributesFormatString=%<BlockChoice>  TemplateBlock=elementsLibrary/propulsion  MemberBlocks=HREV1,SolidMotor
  recovery : Subsystem  BlockChoice=SingleChute
      link override SingleChute: recovery=rocket.recovery
      settings: AttributesFormatString=%<BlockChoice>  TemplateBlock=elementsLibrary/recovery  MemberBlocks=SingleChute
  sequencer : Subsystem  BlockChoice=FSv1
      link override FSv1: sequencer=rocket.sequencer
      settings: AttributesFormatString=%<BlockChoice>  TemplateBlock=elementsLibrary/sequencer  MemberBlocks=FSv1
  acceleration_E : Outport
  angularAcceleration_B : Outport  Port=2
  angularVelocity_B : Outport  Port=3
  position_E : Outport  Port=4
  orientation : Outport  Port=5
  velocity_E : Outport  Port=6
  wires:
  time/1 -> propulsion/1(time)
  Switch/1 -> sequencer/1(position_E), avionics/1(position_E), Unit Delay/1, position_E/1  "position_E"
  Switch1/1 -> avionics/2(orientation), sequencer/2(orientation), orientation/1  "orientation"
  Switch2/1 -> avionics/3(velocity_E), sequencer/3(velocity_E), velocity_E/1  "velocity_E"
  recovery/8(posR_E) -> Switch/1
  recovery/10(velocityR_E) -> Switch2/1
  ascent/4(eulerAngles) -> Switch1/3
  recovery/5(orientationR) -> Switch1/1
  environment/4(Density) -> propulsion/5("density_atm "), ascent/4(density_atm), recovery/2(density_atm)
  environment/6(constants) -> ascent/8(envConstants), recovery/3(envConstants)
  environment/3(Pressure) -> propulsion/4(pressure_atm), ascent/3(pressure_atm)
  environment/2(Temperature) -> propulsion/3(temp_atm), ascent/2(temperature_atm)
  environment/1(windVelocity_E) -> ascent/1(windVelocity_E), recovery/1(windVelocity)
  propulsion/3(propellantMass) -> ascent/16(propellantMass)
  propulsion/1(thrust_B) -> ascent/5(thrust_B), sequencer/4(thrust_B), avionics/4(thrust_B)
  propulsion/5(engineProperties) -> ascent/7(motorProperties)
  propulsion/2(Ve_gas) -> Terminator/1
  sequencer/2(towerVector) -> ascent/10(towerVector)
  ascent/5(angularVelocity) -> recovery/7(inAngVel), Switch4/3
  ascent/1(position_E) -> Switch/3, recovery/6(initPosition_E)
  ascent/2(velocity_E) -> Switch2/3, recovery/5(initVelocity_E)
  recovery/2(angularVelocityP) -> Terminator2/1
  recovery/1(orientationP) -> Terminator1/1
  recovery/3(angularAccelerationP) -> Terminator3/1
  recovery/7(posP_E) -> Terminator4/1
  recovery/9(velocityP_E) -> Terminator5/1
  ascent/3(acceleration_E) -> Switch3/3
  ascent/7(quaternions) -> recovery/4(inQuaternions)
  Demux/3 -> environment/1(altitude_E)
  Demux/2 -> Terminator6/1
  Demux/1 -> Terminator7/1
  recovery/12(accelerationP_E) -> Terminator8/1
  recovery/11(accelerationR_E) -> Switch3/1
  Switch3/1 -> acceleration_E/1  "acceleration_E"
  recovery/4(angularAccelerationR) -> Switch5/1
  recovery/6(angularVelocityR) -> Switch4/1
  ascent/8(angularAcceleration_B) -> Switch5/3
  Switch5/1 -> angularAcceleration_B/1  "angularAcceleration_B"
  Switch4/1 -> angularVelocity_B/1  "angularVelocity_B"
  ascent/6(ddtQuaternions) -> Terminator9/1
  Constant/1 -> ascent/11(rocketEmptyMass)
  Constant1/1 -> ascent/12(rocketEmptyXcg)
  environment/5(kinViscosity_atm) -> ascent/14(kinViscosity_atm)
  avionics/3(descentTwoDeploy) -> recovery/9(descentTwoDeploy), sequencer/6(descentTwoDeploy)
  avionics/2(descentOneDeploy) -> sequencer/5(descentOneDeploy), recovery/8(descentOneDeploy)
  avionics/1(airbrakeCmdAngle) -> ascent/15(airbrakeCmdAngle)
  Unit Delay/1 -> Demux/1
  sequencer/1(flightState) -> ascent/9(flightState), Switch/2, Switch1/2, Switch2/2, Switch4/2, Switch5/2, Switch3/2, recovery/10(flightState)
  propulsion/4(propellantInertias) -> ascent/17(propellantInertias)

== system elementsLibrary/SingleChute ==
  windVelocity : Inport
  density_atm : Inport  Port=2
  envConstants : Inport  Port=3
  inQuaternions : Inport  Port=4
  initVelocity_E : Inport  Port=5
  initPosition_E : Inport  Port=6
  inAngVel : Inport  Port=7
  descentOneDeploy : Inport  Port=8
  descentTwoDeploy : Inport  Port=9
  flightState : Inport  Port=10
  Bus Selector : BusSelector  OutputSignals=M_EARTH,R_EARTH,G_CONST,ANGVEL_EARTH
  Constant : Constant  Value=4
  GreaterThan : RelationalOperator  OutDataTypeStr=boolean  RndMeth=Simplest
  Rotational Motion : Subsystem
  Terminator : Terminator
  Translational Motion : Subsystem
  Unit Delay : UnitDelay  SampleTime=-1
  Unit Delay1 : UnitDelay  SampleTime=-1
  Unit Delay2 : UnitDelay  SampleTime=-1
  orientationP : Outport
  angularVelocityP : Outport  Port=2
  angularAccelerationP : Outport  Port=3
  angularAccelerationR : Outport  Port=4
  orientationR : Outport  Port=5
  angularVelocityR : Outport  Port=6
  posP_E : Outport  Port=7
  posR_E : Outport  Port=8
  velocityP_E : Outport  Port=9
  velocityR_E : Outport  Port=10
  accelerationR_E : Outport  Port=11
  accelerationP_E : Outport  Port=12
  wires:
  Rotational Motion/4(angularAccelerationR) -> angularAccelerationR/1
  Rotational Motion/6(angularVelocityR) -> angularVelocityR/1
  Translational Motion/4(velociyR_E) -> Rotational Motion/3(vR_E), velocityR_E/1
  Rotational Motion/9(quaternions_REP) -> Unit Delay2/1
  Rotational Motion/8(tensionR_E) -> Unit Delay1/1  "tensionRocket_E"
  Translational Motion/3(velocityP_E) -> velocityP_E/1, Rotational Motion/4(vP_E)
  Rotational Motion/3(angularAccelerationP) -> angularAccelerationP/1
  Rotational Motion/1(orientationP) -> orientationP/1
  Rotational Motion/5(orientationR) -> orientationR/1
  Rotational Motion/7(tensionP_E) -> Unit Delay/1  "tensionPrachute_E"
  Rotational Motion/2(angularVelocityP) -> angularVelocityP/1
  windVelocity/1 -> Translational Motion/4(wind_velocity)
  Bus Selector/2 -> Translational Motion/6(R_EARTH)  "<R_EARTH>"
  Bus Selector/1 -> Translational Motion/5(M_EARTH)  "<M_EARTH>"
  Bus Selector/3 -> Translational Motion/7(G_CONST)  "<G_CONST>"
  envConstants/1 -> Bus Selector/1
  density_atm/1 -> Translational Motion/8(density_atm)
  Bus Selector/4 -> Terminator/1  "<ANGVEL_EARTH>"
  inQuaternions/1 -> Rotational Motion/5(initQuaternions)
  initVelocity_E/1 -> Translational Motion/9(initVelocity_E)
  initPosition_E/1 -> Translational Motion/10(initPosition_E)
  inAngVel/1 -> Rotational Motion/6(initAngVel)
  descentOneDeploy/1 -> Translational Motion/11(descentOneDeploy)
  descentTwoDeploy/1 -> Translational Motion/12(descentTwoDeploy)
  flightState/1 -> GreaterThan/1
  Constant/1 -> GreaterThan/2
  GreaterThan/1 -> Translational Motion/Enable, Rotational Motion/Enable
  Translational Motion/5(accelerationR_E) -> accelerationR_E/1
  Translational Motion/6(accelerationP_E) -> accelerationP_E/1
  Translational Motion/1(posP_E) -> posP_E/1, Rotational Motion/2(posP_E)
  Translational Motion/2(posR_E) -> posR_E/1, Rotational Motion/1(posR_E)
  Unit Delay/1 -> Translational Motion/1(tensionP_E)
  Unit Delay1/1 -> Translational Motion/2(tensionR_E)
  Unit Delay2/1 -> Translational Motion/3(quaternions_REP)

== system elementsLibrary/SolidMotor ==
  time : Inport
  1-D Lookup Table : Lookup_n-D  NumberOfTableDimensions=1  BreakpointsForDimension1=propulsion.thrustProfile(1,:)  Table=propulsion.thrustProfile(2,:)  ExtrapMethod=Clip  UseLastTableValue=on  InternalRulePriority=Speed  RndMeth=Simplest  InputSameDT=on
  1-D Lookup Table1 : Lookup_n-D  NumberOfTableDimensions=1  BreakpointsForDimension1=propulsion.massProfile(1,:)  Table=propulsion.massProfile(2,:)  ExtrapMethod=Clip  UseLastTableValue=on  InternalRulePriority=Speed  RndMeth=Simplest  InputSameDT=on
  Add : Sum
  Bus Creator : BusCreator  Inputs=6
  Constant : Constant  Value=0
  Constant1 : Constant  Value=0
  Divide : Product  Inputs=*/
  Dry (empty) Mass : Constant  Value=propulsion.m_dry
  Exit Area of Nozzle : Constant  Value=propulsion.Ae
  Location of Tip of Motor : Constant  Value=propulsion.X_GM
  Mux : Mux  Inputs=3
  Rate Limiter : RateLimiter  RisingSlewLimit=5.0e6  FallingSlewLimit=-5.0e6  SampleTimeMode=inherited
  Subtract : Sum  Inputs=-+
  Terminator : Terminator
  Unit Delay : UnitDelay  SampleTime=-1
  Wet (Full) Mass1 : Constant  Value=propulsion.m_wet
  calculate motor inertia : Subsystem
  initial CoG of motor wrt X_GM : Constant  Value=propulsion.X_CG_full
  initial inner diamter of grain : Constant  Value=propulsion.d_initalgrainInner
  lendth of grain : Constant  Value=propulsion.l_grain
  outer diameter of grain : Constant  Value=propulsion.d_grainOuter
  thrust_B : Outport
  gasExitSpeed : Outport  Port=2
  motorMass : Outport  Port=3
  motorInertias : Outport  Port=4
  motorGeometry : Outport  Port=5
  wires:
  time/1 -> 1-D Lookup Table1/1, 1-D Lookup Table/1
  1-D Lookup Table/1 -> Divide/1, Mux/1
  Constant/1 -> Mux/2
  Constant1/1 -> Mux/3
  Mux/1 -> thrust_B/1  "thrust_B"
  1-D Lookup Table1/1 -> Add/1
  Dry (empty) Mass/1 -> Add/2
  Add/1 -> calculate motor inertia/1(motorMass), motorMass/1, Unit Delay/1, Subtract/1  "motorMass"
  Wet (Full) Mass1/1 -> Terminator/1
  Exit Area of Nozzle/1 -> Bus Creator/1  "Ae"
  initial CoG of motor wrt X_GM/1 -> Bus Creator/3  "x_cg_B"
  Location of Tip of Motor/1 -> Bus Creator/2  "x_gm_B"
  Bus Creator/1 -> motorGeometry/1
  initial inner diamter of grain/1 -> calculate motor inertia/2(grainInnerDia), Bus Creator/4  "d_initialgrainInner"
  outer diameter of grain/1 -> calculate motor inertia/3(grainOuterDia), Bus Creator/5  "d_grainOuter"
  lendth of grain/1 -> calculate motor inertia/4(grainLength), Bus Creator/6  "l_grain"
  Unit Delay/1 -> Subtract/2
  Subtract/1 -> Divide/2  "massFlowRate"
  Divide/1 -> Rate Limiter/1  "noLimVe"
  calculate motor inertia/1(J_motor) -> motorInertias/1  "motorInertias"
  Rate Limiter/1 -> gasExitSpeed/1  "gasExitSpeed"

== system elementsLibrary/aerodynamics ==
  quaternions : Inport
  temperature_atm : Inport  Port=2
  pressure_atm : Inport  Port=3
  density_atm : Inport  Port=4
  windVelocity_B : Inport  Port=5
  kinematicVelocity_B : Inport  Port=6
  kinViscosity_atm : Inport  Port=7
  Xcg : Inport  Port=8
  barrowmanExt : $bdroot/barrowmanExt  aerodynamics=aerodynamics
  moments_B : Outport
  Faero_B : Outport  Port=2
  Xcp : Outport  Port=3
  mach : Outport  Port=4
  wires:
  quaternions/1 -> barrowmanExt/1
  temperature_atm/1 -> barrowmanExt/2
  pressure_atm/1 -> barrowmanExt/3
  density_atm/1 -> barrowmanExt/4
  windVelocity_B/1 -> barrowmanExt/5
  kinematicVelocity_B/1 -> barrowmanExt/6
  kinViscosity_atm/1 -> barrowmanExt/7
  Xcg/1 -> barrowmanExt/8
  barrowmanExt/1 -> moments_B/1
  barrowmanExt/2 -> Faero_B/1
  barrowmanExt/3 -> Xcp/1
  barrowmanExt/4 -> mach/1

== system elementsLibrary/ascent ==
  windVelocity_E : Inport
  temperature_atm : Inport  Port=2
  pressure_atm : Inport  Port=3
  density_atm : Inport  Port=4
  thrust_B : Inport  Port=5
  motorMass : Inport  Port=6
  motorProperties : Inport  Port=7
  envConstants : Inport  Port=8
  flightState : Inport  Port=9
  towerVector : Inport  Port=10
  rocketEmptyMass : Inport  Port=11
  rocketEmptyXcg : Inport  Port=12
  motorInertias : Inport  Port=13
  kinViscosity_atm : Inport  Port=14
  airbrakeCmdAngle : Inport  Port=15
  propellantMass : Inport  Port=16
  propellantInertias : Inport  Port=17
  Ascentv1 : $bdroot/Ascentv1  ascent=ascent
  term16 : Terminator
  term17 : Terminator
  position_E : Outport
  velocity_E : Outport  Port=2
  acceleration_E : Outport  Port=3
  eulerAngles : Outport  Port=4
  angularVelocity : Outport  Port=5
  ddtQuaternions : Outport  Port=6
  quaternions : Outport  Port=7
  angularAcceleration_B : Outport  Port=8
  wires:
  windVelocity_E/1 -> Ascentv1/1
  temperature_atm/1 -> Ascentv1/2
  pressure_atm/1 -> Ascentv1/3
  density_atm/1 -> Ascentv1/4
  thrust_B/1 -> Ascentv1/5
  motorMass/1 -> Ascentv1/6
  motorProperties/1 -> Ascentv1/7
  envConstants/1 -> Ascentv1/8
  flightState/1 -> Ascentv1/9
  towerVector/1 -> Ascentv1/10
  rocketEmptyMass/1 -> Ascentv1/11
  rocketEmptyXcg/1 -> Ascentv1/12
  motorInertias/1 -> Ascentv1/13
  kinViscosity_atm/1 -> Ascentv1/14
  airbrakeCmdAngle/1 -> Ascentv1/15
  Ascentv1/1 -> position_E/1
  Ascentv1/2 -> velocity_E/1
  Ascentv1/3 -> acceleration_E/1
  Ascentv1/4 -> eulerAngles/1
  Ascentv1/5 -> angularVelocity/1
  Ascentv1/6 -> ddtQuaternions/1
  Ascentv1/7 -> quaternions/1
  Ascentv1/8 -> angularAcceleration_B/1
  propellantMass/1 -> term16/1
  propellantInertias/1 -> term17/1

== system elementsLibrary/avionics ==
  position_E : Inport
  orientation : Inport  Port=2
  velocity_E : Inport  Port=3
  thrust_B : Inport  Port=4
  Avionicsv1 : $bdroot/Avionicsv1  avionics=avionics
  airbrakeCmdAngle : Outport
  descentOneDeploy : Outport  Port=2
  descentTwoDeploy : Outport  Port=3
  wires:
  position_E/1 -> Avionicsv1/1
  orientation/1 -> Avionicsv1/2
  velocity_E/1 -> Avionicsv1/3
  thrust_B/1 -> Avionicsv1/4
  Avionicsv1/1 -> airbrakeCmdAngle/1
  Avionicsv1/2 -> descentOneDeploy/1
  Avionicsv1/3 -> descentTwoDeploy/1
